simulink model "pem_electrolyser"  (R2024a)
settings: Solver=VariableStepAuto  StartTime=0.0  StopTime=10.0  RelTol=1e-3
values from neighbouring files (symbols this model uses):
  alpha_a = 0.5    [setup_electrolyzer_params.m]
  alpha_c = 0.5    [setup_electrolyzer_params.m]
  F = 96485.3    [setup_electrolyzer_params.m]
  l_mem = 180e-4    (= 0.018)    [setup_electrolyzer_params.m]
  R = 8.314    [setup_electrolyzer_params.m]
  sigma_mem = (0.005139 * 15 - 0.00326) * exp(1268 * (1/303 - 1/T_op))    [setup_electrolyzer_params.m]
  T_op = 80 + 273.15    (= 353.15)    [setup_electrolyzer_params.m]
  V_rev = E0_T + (R * T_op / (2 * F)) * log(P_H2 * sqrt(P_O2) / P_H2O)    [setup_electrolyzer_params.m]
libraries: simulink x1
settings Model: Creator=Pawan  LastModifiedBy=Pawan

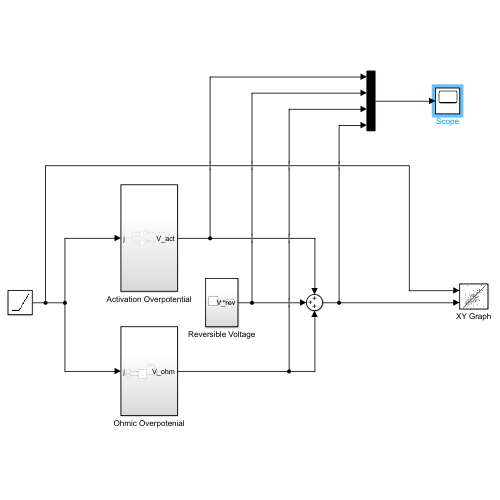
[thumbnail: Simulink's stored preview of the top-level diagram]
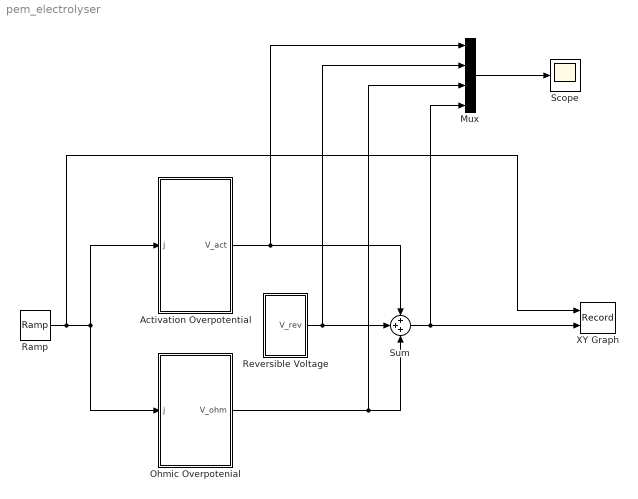
== system pem_electrolyser ==
  Activation Overpotential : Subsystem
  Mux : Mux
  Ohmic Overpotenial : Subsystem
  Ramp : simulink/Sources/Ramp  slope=0.2  start=0  InitialOutput=0
  Reversible Voltage : Subsystem
  Scope : Scope
  Sum : Sum  Inputs=+++
  XY Graph : Record  FileSettingsInternal="{\"entries\":[{\"content\":{\"excelSettings\":{\"content\":{},\"type\":\"Streamout.ExcelSettings\"}},\"type\":\"Streamout.FileSettingStorage\",\"uuid\":\"\"}],\"packageUris\":[\"http:\\/\\/schema.mathworks.com\\/mf0\\/streamout_blocks\\/R2020a\"],\"version\":\"1.0\"}"  Layout=[1 1]  SignalsInternal="{\"entries\":[{\"content\":{\"signals\":[{\"content\":{\"blockPath\":[],\"dimensions\":[1],\"domain\":\"\",\"lineColor\":\"#ff6929\",\"lineWidth\":2,\"plots\":[ 1 ],\"port\":1,\"sid\":[\"\"],\"signalID\":1,\"signalName\":\"Ramp\"},\"type\":\"RecordBlkView.Signal\",\"uuid\":\"\"},{\"content\":{\"blockPath\":[],\"dimensions\":[1],\"domain\":\"\",\"lineColor\":\"#b746ff\",\"lineWidth\":2,\"plots\":[ 1 ],\"port\":2,\"sid\":[\"\"],\"signalID\":2,\"signalName\":\"Sum\"},\"type\":\"RecordBlkView.Signal\",\"uuid\":\"\"}]},\"type\":\"RecordBlkView.InputSignals\",\"uuid\":\"\"}],\"packageUris\":[\"http:\\/\\/schema.mathworks.com\\/mf0\\/streamout_blocks\\/R2020a\"],\"version\":\"1.0\"}"  VisualizationBindings="{\"xyplotplugin\":{\"info\":[{\"series\":[{\"bindingParametersList\":[{\"parameter\":\"X-Axis\",\"signalID\":1,\"signalName\":\"Ramp\"},{\"parameter\":\"Y-Axis\",\"signalID\":2,\"signalName\":\"Sum\"}],\"seriesID\":0}],\"subplotID\":1}]}}"  CompatibilityTag=XY
  wires:
  Ramp/1 -> XY Graph/1, Activation Overpotential/1(j), Ohmic Overpotenial/1(j)
  Sum/1 -> Mux/4, XY Graph/2
  Reversible Voltage/1(V_rev) -> Sum/2, Mux/2
  Ohmic Overpotenial/1(V_ohm) -> Mux/3, Sum/3
  Activation Overpotential/1(V_act) -> Mux/1, Sum/1
  Mux/1 -> Scope/1

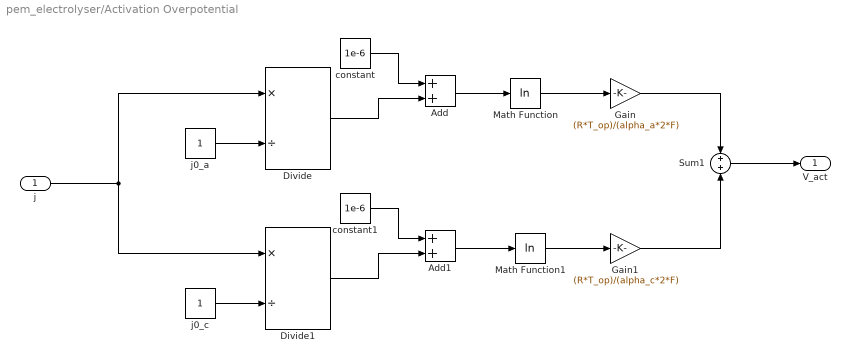
== system pem_electrolyser/Activation Overpotential ==
  j : Inport
  Add : Sum
  Add1 : Sum
  Divide : Product  Inputs=*/
  Divide1 : Product  Inputs=*/
  Gain : Gain  Gain=(R*T_op)/(alpha_a*2*F)
  Gain1 : Gain  Gain=(R*T_op)/(alpha_c*2*F)
  Math Function : Math  Operator=log
  Math Function1 : Math  Operator=log
  Sum1 : Sum
  constant : Constant  Value=1e-6
  constant1 : Constant  Value=1e-6
  j0_a : Constant
  j0_c : Constant
  V_act : Outport
  wires:
  Divide/1 -> Add/2
  Add/1 -> Math Function/1
  Math Function/1 -> Gain/1
  constant/1 -> Add/1
  Divide1/1 -> Add1/2
  constant1/1 -> Add1/1
  Math Function1/1 -> Gain1/1
  Add1/1 -> Math Function1/1
  Gain/1 -> Sum1/1
  Gain1/1 -> Sum1/2
  j0_c/1 -> Divide1/2
  j0_a/1 -> Divide/2
  Sum1/1 -> V_act/1
  j/1 -> Divide/1, Divide1/1

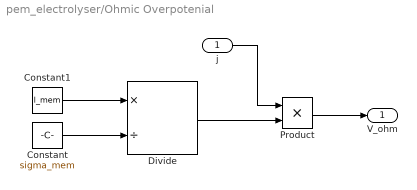
== system pem_electrolyser/Ohmic Overpotenial ==
  j : Inport
  Constant : Constant  Value=sigma_mem
  Constant1 : Constant  Value=l_mem
  Divide : Product  Inputs=*/
  Product : Product
  V_ohm : Outport
  wires:
  Constant1/1 -> Divide/1
  Product/1 -> V_ohm/1
  j/1 -> Product/1
  Divide/1 -> Product/2
  Constant/1 -> Divide/2

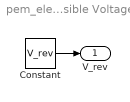
== system pem_electrolyser/Reversible Voltage ==
  Constant : Constant  Value=V_rev
  V_rev : Outport
  wires:
  Constant/1 -> V_rev/1
